simulink model "simu_Lucian2024"  (R2023b)
settings: Solver=VariableStepAuto  StartTime=0.0  StopTime=Tsim  RelTol=1e-3
values from neighbouring files (symbols this model uses):
  A = [-a_til(2:end)' [eye(length(a_til)-2); zeros(1,length(a_til)-2)]]    [Lucian2024.m]    (also in Lucian2024_v2.m; PID_GPC.m = block.DialogPrm(16).Data; QPsolver.m = block.DialogPrm(16).Data)
  B = [b(2:end)']    [Lucian2024.m]    (also in Lucian2024_v2.m)
  D = [c(2:end)'-a_til(2:end)']    [Lucian2024.m]    (also in Lucian2024_v2.m)
  Delta = tf([1 -1],[1],Ts,'Variable','z^-1')    [Lucian2024.m]    (also in Lucian2024_v2.m)
  du_max = 0.5    [Lucian2024.m]    (also in Lucian2024_v2.m; PID_GPC.m = block.DialogPrm(8).Data; QPsolver.m = block.DialogPrm(8).Data)
  du_min = -0.5    [Lucian2024.m]    (also in Lucian2024_v2.m; PID_GPC.m = block.DialogPrm(9).Data; QPsolver.m = block.DialogPrm(9).Data)
  F = block.DialogPrm(1).Data    [PID_GPC.m]    (also in QPsolver.m)
  G = G(:,1:Nu)    [Lucian2024.m]    (also in Lucian2024_v2.m; PID_GPC.m = block.DialogPrm(3).Data; QPsolver.m = block.DialogPrm(3).Data)
  H = [1 zeros(1,Max-1)]    [Lucian2024.m]    (also in Lucian2024_v2.m)
  lambda = 0    [Lucian2024.m]    (also in Lucian2024_v2.m; PID_GPC.m = block.DialogPrm(14).Data; QPsolver.m = block.DialogPrm(14).Data)
  lambda_e = 1000    [Lucian2024.m]    (also in Lucian2024_v2.m; PID_GPC.m = block.DialogPrm(15).Data; QPsolver.m = block.DialogPrm(15).Data)
  N = 20    [Lucian2024.m]    (also in Lucian2024_v2.m; PID_GPC.m = block.DialogPrm(11).Data; QPsolver.m = block.DialogPrm(11).Data)
  Nu = 1    [Lucian2024.m]    (also in Lucian2024_v2.m; PID_GPC.m = block.DialogPrm(12).Data; QPsolver.m = block.DialogPrm(12).Data)
  pert = -0.1    [Lucian2024.m]    (also in Lucian2024_v2.m)
  Q = eye(N)    [Lucian2024.m]    (also in Lucian2024_v2.m; PID_GPC.m = block.DialogPrm(13).Data; QPsolver.m = block.DialogPrm(13).Data)
  r1 = 0.5    [Lucian2024.m]    (also in Lucian2024_v2.m)
  r2 = 0.3    [Lucian2024.m]    (also in Lucian2024_v2.m)
  Tpert = ceil(30/Ts)    [Lucian2024.m]    (also in Lucian2024_v2.m)
  Tr1 = ceil(1/Ts)    [Lucian2024.m]    (also in Lucian2024_v2.m)
  Tr2 = ceil(45/Ts)    [Lucian2024.m]    (also in Lucian2024_v2.m)
  Ts = 0.1    [Lucian2024.m]    (also in Lucian2024_v2.m; PID_GPC.m = block.DialogPrm(10).Data; QPsolver.m = block.DialogPrm(10).Data)
  u_max = 0.9    [Lucian2024.m]    (also in Lucian2024_v2.m; PID_GPC.m = block.DialogPrm(6).Data; QPsolver.m = block.DialogPrm(6).Data)
  u_min = 0    [Lucian2024.m]    (also in Lucian2024_v2.m; PID_GPC.m = block.DialogPrm(7).Data; QPsolver.m = block.DialogPrm(7).Data)
  y_max = 0.7    [Lucian2024.m]    (also in Lucian2024_v2.m; PID_GPC.m = block.DialogPrm(4).Data; QPsolver.m = block.DialogPrm(4).Data)
  y_min = 0    [Lucian2024.m]    (also in Lucian2024_v2.m; PID_GPC.m = block.DialogPrm(5).Data; QPsolver.m = block.DialogPrm(5).Data)
libraries: cstblocks x8
settings Model: Creator=sergio  LastModifiedBy=sergio

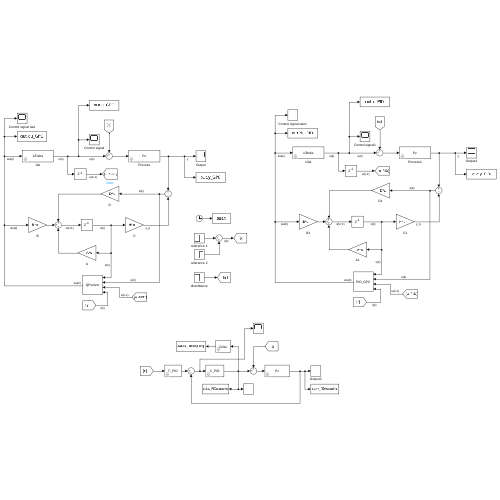
[thumbnail: Simulink's stored preview of the top-level diagram]
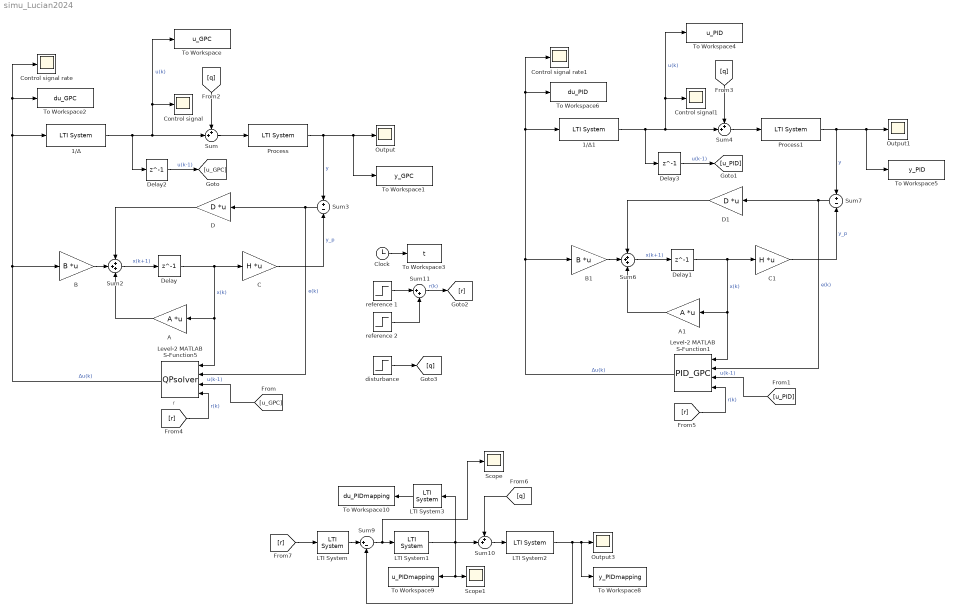
== system simu_Lucian2024 ==
  note: r
  1/Δ : cstblocks/LTI System  sys=1/Delta  IC=[]  PadeOrder=0
  1/Δ1 : cstblocks/LTI System  sys=1/Delta  IC=[]  PadeOrder=0
  A : Gain  Gain=A  Multiplication=Matrix(K*u)
  A1 : Gain  Gain=A  Multiplication=Matrix(K*u)
  B : Gain  Gain=B  Multiplication=Matrix(K*u)
  B1 : Gain  Gain=B  Multiplication=Matrix(K*u)
  C : Gain  Gain=H  Multiplication=Matrix(K*u)
  C1 : Gain  Gain=H  Multiplication=Matrix(K*u)
  Clock : Clock
  Control signal : Scope
  Control signal rate : Scope
  Control signal rate1 : Scope
  Control signal1 : Scope
  D : Gain  Gain=D  Multiplication=Matrix(K*u)
  D1 : Gain  Gain=D  Multiplication=Matrix(K*u)
  Delay{,1..3} (4 alike) : Delay  DelayLength=1  SampleTime=Ts
  LTI System : cstblocks/LTI System  sys=F_PID  IC=[]  PadeOrder=0
  LTI System1 : cstblocks/LTI System  sys=C_PID  IC=[]  PadeOrder=0
  LTI System2 : cstblocks/LTI System  sys=Pz  IC=[]  PadeOrder=0
  LTI System3 : cstblocks/LTI System  sys=Delta  IC=[]  PadeOrder=0
  Level-2 MATLAB S-Function1 : M-S-Function  FunctionName=PID_GPC  Parameters=F,E,G,y_max,y_min,u_max,u_min,du_max,du_min,Ts,N,Nu,Q,lambda,lambda_e,A
  Level-2 MATLAB S-Function5 : M-S-Function  FunctionName=QPsolver  Parameters=F,E,G,y_max,y_min,u_max,u_min,du_max,du_min,Ts,N,Nu,Q,lambda,lambda_e,A
  Output : Scope
  Output1 : Scope
  Output3 : Scope
  Process : cstblocks/LTI System  sys=Pz  IC=[]  PadeOrder=0
  Process1 : cstblocks/LTI System  sys=Pz  IC=[]  PadeOrder=0
  Scope : Scope
  Scope1 : Scope
  Sum : Sum  Inputs=++|
  Sum10 : Sum  Inputs=++|
  Sum11 : Sum  Inputs=|++
  Sum2 : Sum  Inputs=+++
  Sum3 : Sum  Inputs=+|-
  Sum4 : Sum  Inputs=++|
  Sum6 : Sum  Inputs=+++
  Sum7 : Sum  Inputs=+|-
  Sum9 : Sum  Inputs=|+-
  To Workspace : ToWorkspace  VariableName=u_GPC  SampleTime=Ts
      settings: Save2DSignal=2-D array (concatenate along first dimension)
  To Workspace1 : ToWorkspace  VariableName=y_GPC  SampleTime=Ts
      settings: Save2DSignal=2-D array (concatenate along first dimension)
  To Workspace10 : ToWorkspace  VariableName=du_PIDmapping  SampleTime=Ts
  To Workspace2 : ToWorkspace  VariableName=du_GPC  SampleTime=Ts
      settings: Save2DSignal=2-D array (concatenate along first dimension)
  To Workspace3 : ToWorkspace  VariableName=t  SampleTime=Ts
      settings: Save2DSignal=2-D array (concatenate along first dimension)
  To Workspace4 : ToWorkspace  VariableName=u_PID  SampleTime=Ts
      settings: Save2DSignal=2-D array (concatenate along first dimension)
  To Workspace5 : ToWorkspace  VariableName=y_PID  SampleTime=Ts
      settings: Save2DSignal=2-D array (concatenate along first dimension)
  To Workspace6 : ToWorkspace  VariableName=du_PID  SampleTime=Ts
      settings: Save2DSignal=2-D array (concatenate along first dimension)
  To Workspace8 : ToWorkspace  VariableName=y_PIDmapping  SampleTime=Ts
  To Workspace9 : ToWorkspace  VariableName=u_PIDmapping  SampleTime=Ts
  disturbance : Step  Time=Tpert*Ts  After=pert  SampleTime=Ts
  reference 1 : Step  Time=Tr1*Ts  After=r1  SampleTime=Ts
  reference 2 : Step  Time=Tr2*Ts  After=r2  SampleTime=Ts
  wires:
  [q] -> Sum/1
  B/1 -> Sum2/2
  Level-2 MATLAB S-Function5/1 -> To Workspace2/1, Control signal rate/1, 1/Δ/1, B/1  "Δu(k)"
  C/1 -> Sum3/2  "y_p"
  A/1 -> Sum2/3
  Sum2/1 -> Delay/1  "x(k+1)"
  Sum/1 -> Process/1
  1/Δ/1 -> Delay2/1, To Workspace/1, Control signal/1, Sum/2  "u(k)"
  [u_GPC] -> Level-2 MATLAB S-Function5/3  "u(k-1)"
  Delay2/1 -> [u_GPC]  "u(k-1)"
  Delay/1 -> Level-2 MATLAB S-Function5/1, A/1, C/1  "x(k)"
  Sum3/1 -> Level-2 MATLAB S-Function5/2, D/1  "e(k)"
  Process/1 -> To Workspace1/1, Output/1, Sum3/1  "y"
  D/1 -> Sum2/1
  [r] -> Level-2 MATLAB S-Function5/4  "r(k)"
  Clock/1 -> To Workspace3/1
  Level-2 MATLAB S-Function1/1 -> Control signal rate1/1, To Workspace6/1, 1/Δ1/1, B1/1  "Δu(k)"
  Delay3/1 -> [u_PID]  "u(k-1)"
  Process1/1 -> To Workspace5/1, Output1/1, Sum7/1  "y"
  [r] -> Level-2 MATLAB S-Function1/4  "r(k)"
  Sum7/1 -> D1/1, Level-2 MATLAB S-Function1/2  "e(k)"
  [q] -> Sum4/1
  1/Δ1/1 -> Delay3/1, To Workspace4/1, Control signal1/1, Sum4/2  "u(k)"
  [u_PID] -> Level-2 MATLAB S-Function1/3  "u(k-1)"
  Sum4/1 -> Process1/1
  B1/1 -> Sum6/2
  A1/1 -> Sum6/3
  C1/1 -> Sum7/2  "y_p"
  Delay1/1 -> Level-2 MATLAB S-Function1/1, A1/1, C1/1  "x(k)"
  Sum6/1 -> Delay1/1  "x(k+1)"
  D1/1 -> Sum6/1
  Sum10/1 -> LTI System2/1
  [q] -> Sum10/1
  LTI System/1 -> Sum9/1
  [r] -> LTI System/1
  LTI System2/1 -> Sum9/2, To Workspace8/1, Output3/1
  LTI System1/1 -> Scope1/1, To Workspace9/1, LTI System3/1, Sum10/2
  LTI System3/1 -> To Workspace10/1
  reference 1/1 -> Sum11/1
  reference 2/1 -> Sum11/2
  Sum11/1 -> [r]  "r(k)"
  disturbance/1 -> [q]
  Sum9/1 -> Scope/1, LTI System1/1
